simulink model "ship_5_5_e_old"  (Simulink 8.5)
settings: Solver=ode45  StartTime=0.0  StopTime=500  RelTol=1e-3
values from neighbouring files (symbols this model uses):
  psi_r = 30    [problem3.m]    (also in problem5.m)
  Ts = 1/10    (= 0.1)    [problem5.m]
libraries: simeventslib x4, simulink x2, cstblocks x1
settings Model: Creator=markh  LastModifiedBy=martinty
settings SolverCC: AlgebraicLoopSolver=LineSearch
settings DataIOCC: SignalLoggingName=sigsOut
settings OptimizationCC: ExpressionDepthLimit=128  InitFltsAndDblsToZero=on
settings DebuggingCC: SaveWithParameterizedLinksMsg=none  SignalResolutionControl=TryResolveAllWithWarning  MultiTaskDSMMsg=warning  MultiTaskCondExecSysMsg=none  FcnCallInpInsideContextMsg=UseLocalSettings
settings HardwareCC: TargetUnknown=on
settings GRTTargetCC: TargetFcnLib=ansi_tfl_tmw.mat

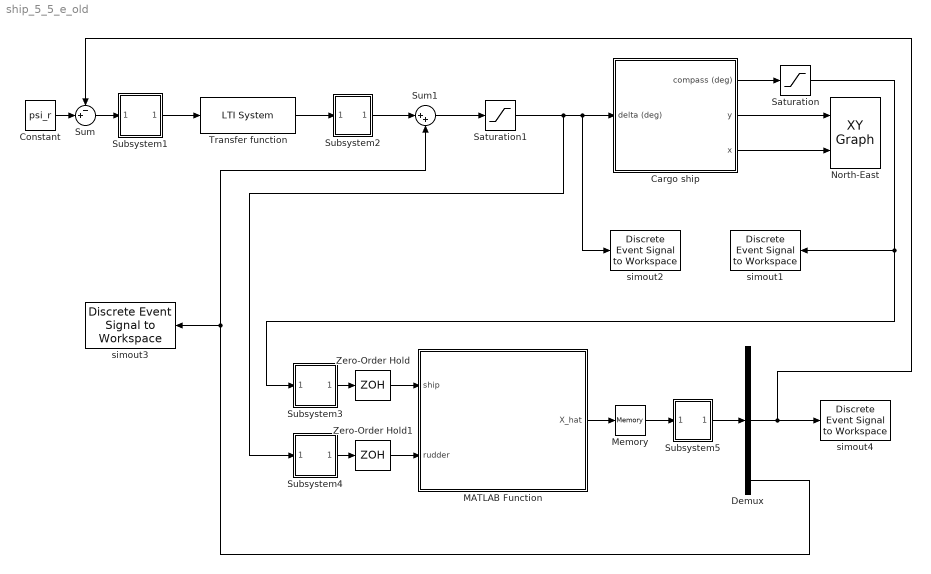
== system ship_5_5_e_old ==
  Cargo ship : Subsystem  mask(Simple shipmodel for a cargo ship){noise=on, current=on, logic=on}
      mask prompts: noise "measurement noise"; logic "waves"
      mask help:
      | Measurement noise:
      | 	checked = noise on
      | 	unchecked = noise off
      |
      | Current:
      | 	checked = current on
      | 	unchecked = current off
      |
      | Waves:
      | 	checked = waves on
      | 	unchecked = waves off
      |
      | Author: Jørgen Spjøtvold, 9/10-2003
      | TTK 4115 Linear system theory.
      | Modified by Jostein Bakkeheim 26/10-2006
  Constant : Constant  Value=psi_r
  Demux : Demux  Outputs=5
  MATLAB Function : MATLAB Function  TreatAsAtomicUnit=on
  Memory : Memory
  North-East : simulink/Sinks/XY Graph  xmin=-5000  xmax=5000  ymin=-5000  ymax=5000  st=-1
  Saturation : Saturate  UpperLimit=35  LowerLimit=-35
  Saturation1 : Saturate  UpperLimit=45  LowerLimit=-45
  Subsystem1 : Subsystem  mask(degrees to radians){}
      mask help: Converts degrees to radians
      mask Display: fprintf('D2R');
  Subsystem2 : Subsystem  mask(radians to degrees){}
      mask help: Converts radians to degrees
      mask Display: fprintf('R2D');
  Subsystem3 : Subsystem  mask(degrees to radians){}
      mask help: Converts degrees to radians
      mask Display: fprintf('D2R');
  Subsystem4 : Subsystem  mask(degrees to radians){}
      mask help: Converts degrees to radians
      mask Display: fprintf('D2R');
  Subsystem5 : Subsystem  mask(radians to degrees){}
      mask help: Converts radians to degrees
      mask Display: fprintf('R2D');
  Sum : Sum  Inputs=-+|
  Sum1 : Sum  Inputs=|++
  Transfer function : cstblocks/LTI System  sys=H_pd  IC=[]
  Zero-Order Hold : ZeroOrderHold  SampleTime=Ts
  Zero-Order Hold1 : ZeroOrderHold  SampleTime=Ts
  simout1 : simeventslib/SimEvents Sinks/Discrete Event Signal to Workspace  VariableName=ship  SaveFormat=Structure With Time  isMonitorOnly=off  isRecordIC=off
  simout2 : simeventslib/SimEvents Sinks/Discrete Event Signal to Workspace  VariableName=rudder  SaveFormat=Structure With Time  isMonitorOnly=off  isRecordIC=off
  simout3 : simeventslib/SimEvents Sinks/Discrete Event Signal to Workspace  VariableName=bias_estimate  SaveFormat=Structure With Time  isMonitorOnly=off  isRecordIC=off
  simout4 : simeventslib/SimEvents Sinks/Discrete Event Signal to Workspace  VariableName=ship_estimate  SaveFormat=Structure With Time  isMonitorOnly=off  isRecordIC=off
  wires:
  Cargo ship/3(x) -> North-East/2
  Cargo ship/2(y) -> North-East/1
  Cargo ship/1(compass (deg)) -> Saturation/1
  Saturation/1 -> simout1/1, Subsystem3/1(In1)
  Subsystem1/1(Out1) -> Transfer function/1
  Sum/1 -> Subsystem1/1(In1)
  Saturation1/1 -> simout2/1, Cargo ship/1(delta (deg)), Subsystem4/1(In1)
  Constant/1 -> Sum/2
  Zero-Order Hold/1 -> MATLAB Function/1(ship)
  Zero-Order Hold1/1 -> MATLAB Function/2(rudder)
  MATLAB Function/1(X_hat) -> Memory/1
  Memory/1 -> Subsystem5/1(In1)
  Transfer function/1 -> Subsystem2/1(In1)
  Subsystem2/1(Out1) -> Sum1/1
  Sum1/1 -> Saturation1/1
  Demux/5 -> Sum1/2, simout3/1
  Subsystem3/1(Out1) -> Zero-Order Hold/1
  Subsystem4/1(Out1) -> Zero-Order Hold1/1
  Subsystem5/1(Out1) -> Demux/1
  Demux/3 -> simout4/1, Sum/1

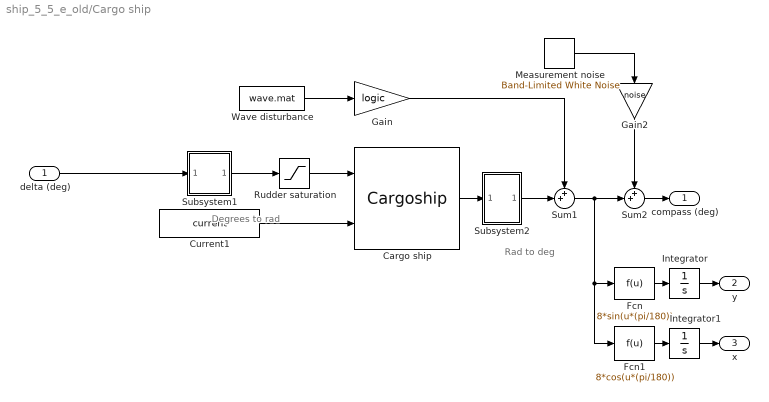
== system ship_5_5_e_old/Cargo ship ==
  note: Degrees to rad
  note: Rad to deg
  delta (deg) : Inport
  Cargo ship : S-Function  FunctionName=Cargoship  mask(Cargo ship){}
      mask help:
      | S-function which simulates a cargo ship.
      |
      | Author: Jørgen Spjøtvold
      | 20.10-2003
      | Modified by Jostein Bakkeheim 27.10.2006
  Current1 : Constant  Value=current
  Fcn : Fcn  Expr=8*sin(u*(pi/180))
  Fcn1 : Fcn  Expr=8*cos(u*(pi/180))
  Gain : Gain  Gain=logic  SaturateOnIntegerOverflow=on  OutDataTypeStr=Inherit: Same as input  ParamDataTypeStr=Inherit: Same as input
  Gain2 : Gain  Gain=noise  SaturateOnIntegerOverflow=on  OutDataTypeStr=Inherit: Same as input  ParamDataTypeStr=Inherit: Same as input
  Integrator : Integrator
  Integrator1 : Integrator
  Measurement noise : simulink/Sources/Band-Limited White Noise  Cov=[0.001]  Ts=.5  seed=[23341]
  Rudder saturation : Saturate  UpperLimit=45*(pi/180)  LowerLimit=-45*(pi/180)
  Subsystem1 : Subsystem  mask(degrees to radians){}
      mask help: Converts degrees to radians
      mask Display: fprintf('D2R');
  Subsystem2 : Subsystem  mask(radians to degrees){}
      mask help: Converts radians to degrees
      mask Display: fprintf('R2D');
  Sum1 : Sum  Inputs=++|  SaturateOnIntegerOverflow=on
  Sum2 : Sum  Inputs=++|  SaturateOnIntegerOverflow=on
  Wave disturbance : FromFile  FileName=wave.mat  SampleTime=0
  compass (deg) : Outport
  y : Outport  Port=2
  x : Outport  Port=3
  wires:
  Fcn/1 -> Integrator/1
  Integrator/1 -> y/1
  Fcn1/1 -> Integrator1/1
  Integrator1/1 -> x/1
  Wave disturbance/1 -> Gain/1
  Subsystem2/1(Out1) -> Sum1/2
  Sum1/1 -> Fcn/1, Fcn1/1, Sum2/2
  Cargo ship/1 -> Subsystem2/1(In1)
  Subsystem1/1(Out1) -> Rudder saturation/1
  Rudder saturation/1 -> Cargo ship/1
  Sum2/1 -> compass (deg)/1
  Measurement noise/1 -> Gain2/1
  Current1/1 -> Cargo ship/2
  Gain/1 -> Sum1/1
  Gain2/1 -> Sum2/1
  delta (deg)/1 -> Subsystem1/1(In1)

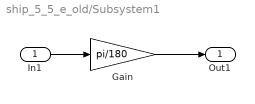
== system ship_5_5_e_old/Subsystem1 ==
  In1 : Inport
  Gain : Gain  Gain=pi/180  SaturateOnIntegerOverflow=on  OutDataTypeStr=Inherit: Same as input  ParamDataTypeStr=Inherit: Same as input
  Out1 : Outport
  wires:
  Gain/1 -> Out1/1
  In1/1 -> Gain/1

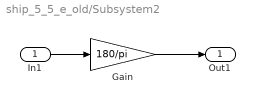
== system ship_5_5_e_old/Subsystem2 ==
  In1 : Inport
  Gain : Gain  Gain=180/pi  SaturateOnIntegerOverflow=on  OutDataTypeStr=Inherit: Same as input  ParamDataTypeStr=Inherit: Same as input
  Out1 : Outport
  wires:
  Gain/1 -> Out1/1
  In1/1 -> Gain/1

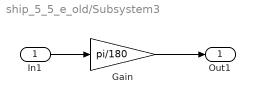
== system ship_5_5_e_old/Subsystem3 ==
  In1 : Inport
  Gain : Gain  Gain=pi/180  SaturateOnIntegerOverflow=on  OutDataTypeStr=Inherit: Same as input  ParamDataTypeStr=Inherit: Same as input
  Out1 : Outport
  wires:
  Gain/1 -> Out1/1
  In1/1 -> Gain/1

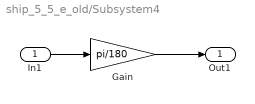
== system ship_5_5_e_old/Subsystem4 ==
  In1 : Inport
  Gain : Gain  Gain=pi/180  SaturateOnIntegerOverflow=on  OutDataTypeStr=Inherit: Same as input  ParamDataTypeStr=Inherit: Same as input
  Out1 : Outport
  wires:
  Gain/1 -> Out1/1
  In1/1 -> Gain/1

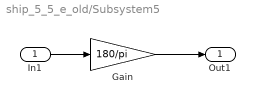
== system ship_5_5_e_old/Subsystem5 ==
  In1 : Inport
  Gain : Gain  Gain=180/pi  SaturateOnIntegerOverflow=on  OutDataTypeStr=Inherit: Same as input  ParamDataTypeStr=Inherit: Same as input
  Out1 : Outport
  wires:
  Gain/1 -> Out1/1
  In1/1 -> Gain/1

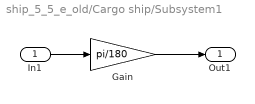
== system ship_5_5_e_old/Cargo ship/Subsystem1 ==
  In1 : Inport
  Gain : Gain  Gain=pi/180  SaturateOnIntegerOverflow=on  OutDataTypeStr=Inherit: Same as input  ParamDataTypeStr=Inherit: Same as input
  Out1 : Outport
  wires:
  Gain/1 -> Out1/1
  In1/1 -> Gain/1

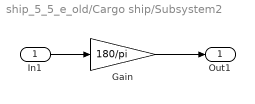
== system ship_5_5_e_old/Cargo ship/Subsystem2 ==
  In1 : Inport
  Gain : Gain  Gain=180/pi  SaturateOnIntegerOverflow=on  OutDataTypeStr=Inherit: Same as input  ParamDataTypeStr=Inherit: Same as input
  Out1 : Outport
  wires:
  Gain/1 -> Out1/1
  In1/1 -> Gain/1

== matlab function MATLAB Function ==
  data: ship input double; X_hat output double; rudder input double; kalmanFilter parameter double
function X_hat = fcn(ship, rudder, kalmanFilter)

persistent P_k X_k init_flag R_rad Q A_d B_d C_d E_d;

if isempty(init_flag)
    init_flag = 1;
    P_k = kalmanFilter.P_0;
    X_k = kalmanFilter.X_0;
    R_rad = kalmanFilter.R_rad;
    Q = kalmanFilter.Q;
    A_d = kalmanFilter.A_d;
    B_d = kalmanFilter.B_d;
    C_d = kalmanFilter.C_d;
    E_d = kalmanFilter.E_d;
end

%(1) Kalman gain
K_k = P_k*C_d'*inv(C_d*P_k*C_d'+R_rad);
%(2) Update estimate
X_hat = X_k + K_k*(ship-C_d*X_k);
%(3) Update covariance
P_k = (eye(5)-K_k*C_d)*P_k*(eye(5)-K_k*C_d)' + K_k*R_rad*K_k';
%(4) Project ahead
X_k = A_d*X_hat + B_d*rudder; 
P_k = A_d*P_k*A_d'+E_d*Q*E_d';

end
